simulink model "PIL_NO_RPI_new"  (R2021a)
settings: Solver=FixedStepAuto  StartTime=0.0  StopTime=60  FixedStep=0.001  RelTol=1e-3  EnableMultiTasking=on
values from neighbouring files (symbols this model uses):
  den_lpf_d = den_lpf20    [Mainframe_init.m]    (also in load_autopilot.m)
  Enable_Gyros = 0    [Mainframe_init.m]
  Enable_INS = 0    [Mainframe_init.m]
  num_lpf_d = num_lpf20    [Mainframe_init.m]    (also in load_autopilot.m)
undefined symbols (not defined in the file or in its folder): act_dmp, act_omega, Actuator, Aerodynamics, aMode, Autopilot, AUX, c_b_WGS, c_be, c_flat, c_grav, c_h_geop0, c_h_geope, c_pa0, c_pe, c_r0, c_rot, c_rsma, c_Tmp0, d_siB_0, d_siB_max, d_siB_min, dd_siB_max, dd_siB_min, dev, DiscIntNeverNeededParam, e_pa, e_Tmp, fin_maxrate, flag_I_act_switch, flag_I_aero_switch, flag_I_flat, flag_I_gravity_switch, flag_I_rot, h_bkpts_m, hcr, HIL_Data, JMMM_0, JMMM_e, JSPB_e, Ki_phi_vec, Kp_p_vec, Kp_phi_vec, lat_0, lon_0, Mass_Props, mB_0, mM_0, mM_e, National_Instruments, Newton, p, pBII_0, PCIe, phi, pMPB, pNPB, propellant_kg, prp_FBPB, prp_mdot ... (+40)
libraries: simulink x32, simulink_extras x23, aerolibcommonsys x4, pil_lib x2, custom_blocks x1, px4lib x1, sldrtlib x1, aerolibnav x1
(part 16 of 16)

== system PIL_NO_RPI_new/Non-linear Flight Dynamic Model1/Subsystem1/GRM_Airframe/motion_kinematics/calc_motion_kinematics/earth_rotation/quaternion_integration/Subsystem1/conjugate_quaternion1 ==
  note: Outputs [size]:
      |
      | q_conj [4]
  note: Inputs [size]:
      |
      | q [4]
  q : Inport
  Demux : Demux  Outputs=[3;1]
  Gain1 : Gain  Gain=-1
  Vector Concatenate : Concatenate
  q_conj : Outport  VectorParamsAs1DForOutWhenUnconnected=off
  wires:
  Demux/2 -> Vector Concatenate/2
  Gain1/1 -> Vector Concatenate/1
  Demux/1 -> Gain1/1
  Vector Concatenate/1 -> q_conj/1
  q/1 -> Demux/1

== system PIL_NO_RPI_new/Non-linear Flight Dynamic Model1/Subsystem1/GRM_Airframe/motion_kinematics/calc_motion_kinematics/earth_rotation/quaternion_integration/Subsystem1/conjugate_quaternion2 ==
  note: Outputs [size]:
      |
      | q_conj [4]
  note: Inputs [size]:
      |
      | q [4]
  q : Inport
  Demux : Demux  Outputs=[3;1]
  Gain1 : Gain  Gain=-1
  Vector Concatenate : Concatenate
  q_conj : Outport  VectorParamsAs1DForOutWhenUnconnected=off
  wires:
  Demux/2 -> Vector Concatenate/2
  Gain1/1 -> Vector Concatenate/1
  Demux/1 -> Gain1/1
  Vector Concatenate/1 -> q_conj/1
  q/1 -> Demux/1

== system PIL_NO_RPI_new/Non-linear Flight Dynamic Model1/Subsystem1/GRM_Airframe/motion_kinematics/calc_motion_kinematics/earth_rotation/quaternion_integration1/Subsystem1/conjugate_quaternion1 ==
  note: Outputs [size]:
      |
      | q_conj [4]
  note: Inputs [size]:
      |
      | q [4]
  q : Inport
  Demux : Demux  Outputs=[3;1]
  Gain1 : Gain  Gain=-1
  Vector Concatenate : Concatenate
  q_conj : Outport  VectorParamsAs1DForOutWhenUnconnected=off
  wires:
  Demux/2 -> Vector Concatenate/2
  Gain1/1 -> Vector Concatenate/1
  Demux/1 -> Gain1/1
  Vector Concatenate/1 -> q_conj/1
  q/1 -> Demux/1

== system PIL_NO_RPI_new/Non-linear Flight Dynamic Model1/Subsystem1/GRM_Airframe/motion_kinematics/calc_motion_kinematics/earth_rotation/quaternion_integration1/Subsystem1/conjugate_quaternion2 ==
  note: Outputs [size]:
      |
      | q_conj [4]
  note: Inputs [size]:
      |
      | q [4]
  q : Inport
  Demux : Demux  Outputs=[3;1]
  Gain1 : Gain  Gain=-1
  Vector Concatenate : Concatenate
  q_conj : Outport  VectorParamsAs1DForOutWhenUnconnected=off
  wires:
  Demux/2 -> Vector Concatenate/2
  Gain1/1 -> Vector Concatenate/1
  Demux/1 -> Gain1/1
  Vector Concatenate/1 -> q_conj/1
  q/1 -> Demux/1

== system PIL_NO_RPI_new/Non-linear Flight Dynamic Model1/Subsystem1/GRM_Airframe/rb_eom/eom_6dof/Rigid_Body_EOM_6_DOF/rb_eom_6dof/calc_d_qIB/conjugate_quaternion ==
  note: Outputs [size]:
      |
      | q_conj [4]
  note: Inputs [size]:
      |
      | q [4]
  q : Inport
  Demux : Demux  Outputs=[3;1]
  Gain1 : Gain  Gain=-1
  Vector Concatenate : Concatenate
  q_conj : Outport  VectorParamsAs1DForOutWhenUnconnected=off
  wires:
  Demux/2 -> Vector Concatenate/2
  Gain1/1 -> Vector Concatenate/1
  Demux/1 -> Gain1/1
  Vector Concatenate/1 -> q_conj/1
  q/1 -> Demux/1

== system PIL_NO_RPI_new/Non-linear Flight Dynamic Model1/Subsystem1/GRM_Airframe/rb_eom/eom_6dof/Rigid_Body_EOM_6_DOF/rb_eom_6dof/calc_d_qIB/conjugate_quaternion1 ==
  note: Outputs [size]:
      |
      | q_conj [4]
  note: Inputs [size]:
      |
      | q [4]
  q : Inport
  Demux : Demux  Outputs=[3;1]
  Gain1 : Gain  Gain=-1
  Vector Concatenate : Concatenate
  q_conj : Outport  VectorParamsAs1DForOutWhenUnconnected=off
  wires:
  Demux/2 -> Vector Concatenate/2
  Gain1/1 -> Vector Concatenate/1
  Demux/1 -> Gain1/1
  Vector Concatenate/1 -> q_conj/1
  q/1 -> Demux/1

== system PIL_NO_RPI_new/Non-linear Flight Dynamic Model1/Subsystem1/GRM_Airframe/aerodynamics/aerodynamic_via_lookup/calc_aero_for_mom/launch_rail/initial_altitude/trafo_E_to_geodetic/Geodetic_altitude ==
  pBEE : Inport
  c_rsma : Inport  Port=2
  c_flat : Inport  Port=3
  lat : Inport  Port=4
  Add : Sum
  Constant : Constant
  Gain : Gain  Gain=2
  Product : Product  Inputs=*/  InputSameDT=on  RndMeth=Zero  SaturateOnIntegerOverflow=on  OutDataTypeStr=Inherit: Same as first input
  Product1 : Product
  Product2 : Product
  Product3 : Product
  Product4 : Product  Inputs=*/  InputSameDT=on  RndMeth=Zero  SaturateOnIntegerOverflow=on  OutDataTypeStr=Inherit: Same as first input
  Product5 : Product  Inputs=3
  Selector : Selector  IndexMode=Zero-based  InputPortWidth=3  IndexOptions=Index vector (dialog)  Indices=0  OutputSizes=1
  Selector1 : Selector  IndexMode=Zero-based  InputPortWidth=3  IndexOptions=Index vector (dialog)  Indices=1  OutputSizes=1
  Sqrt : Sqrt  SaturateOnIntegerOverflow=on
  Sqrt1 : Sqrt  SaturateOnIntegerOverflow=on
  Subtract : Sum  Inputs=+-
  Subtract1 : Sum  Inputs=+-
  Sum : Sum  Inputs=+-  InputSameDT=on  SaturateOnIntegerOverflow=on  OutDataTypeStr=Inherit: Same as first input
  Trigonometric Function : Trigonometry
  cos(latGD) : Trigonometry  Operator=cos
  alt : Outport  VectorParamsAs1DForOutWhenUnconnected=off
  wires:
  Product4/1 -> Sum/2
  Trigonometric Function/1 -> Product5/1, Product5/2
  Product5/1 -> Subtract1/2
  Constant/1 -> Subtract1/1
  Subtract1/1 -> Sqrt1/1
  Sqrt1/1 -> Product4/2
  c_flat/1 -> Gain/1, Product3/2, Product3/1
  Gain/1 -> Subtract/1
  Product3/1 -> Subtract/2
  pBEE/1 -> Selector/1, Selector1/1
  Add/1 -> Sqrt/1
  Product2/1 -> Add/2
  Product1/1 -> Add/1
  Selector1/1 -> Product2/1, Product2/2
  Selector/1 -> Product1/1, Product1/2
  Sum/1 -> alt/1  "alt"
  Product/1 -> Sum/1
  Subtract/1 -> Product5/3
  c_rsma/1 -> Product4/1
  cos(latGD)/1 -> Product/2
  Sqrt/1 -> Product/1
  lat/1 -> cos(latGD)/1, Trigonometric Function/1

== system PIL_NO_RPI_new/Non-linear Flight Dynamic Model1/Subsystem1/GRM_Airframe/aerodynamics/aerodynamic_via_lookup/calc_aero_for_mom/launch_rail/initial_altitude/trafo_E_to_geodetic/Geodetic_latitude ==
  pBEE : Inport
  c_rsma : Inport  Port=2
  c_flat : Inport  Port=3
  Add : Sum
  Add1 : Sum
  Constant : Constant
  Demux1 : Demux  Outputs=[1;1;1]
      settings: DisplayOption=none
  Divide : Product  Inputs=*/
  Divide1 : Product  Inputs=*/
  Divide2 : Product  Inputs=*/
  Gain : Gain  Gain=2
  Product{,1..7} (8 alike) : Product
  Product{8..11} (4 alike) : Product  Inputs=3
  Sqrt : Sqrt  SaturateOnIntegerOverflow=on
  Subtract{,1..3} (4 alike) : Sum  Inputs=+-
  Trigonometric Function : Trigonometry  Operator=atan
  Trigonometric Function1 : Trigonometry  Operator=atan
  Trigonometric Function2 : Trigonometry
  Trigonometric Function3 : Trigonometry  Operator=cos
  lat : Outport  VectorParamsAs1DForOutWhenUnconnected=off
  wires:
  Divide/1 -> Product10/1
  Product9/1 -> Product11/3
  Product11/1 -> Subtract3/2
  Subtract3/1 -> Divide2/2
  Add1/1 -> Divide2/1
  Product10/1 -> Add1/2
  Product8/1 -> Product10/3
  Trigonometric Function3/1 -> Product9/1, Product9/3, Product9/2
  Trigonometric Function2/1 -> Product8/1, Product8/3, Product8/2
  Divide2/1 -> Trigonometric Function1/1
  Divide1/1 -> Trigonometric Function/1
  Product7/1 -> Divide1/2
  Product6/1 -> Divide1/1
  Subtract2/1 -> Divide/1
  Product5/1 -> Divide/2, Subtract2/2
  Product4/1 -> Subtract2/1
  Gain/1 -> Subtract1/1
  Product3/1 -> Subtract1/2
  Sqrt/1 -> [P]
  Add/1 -> Sqrt/1
  Product2/1 -> Add/2
  Product1/1 -> Add/1
  Product/1 -> [b]
  Subtract/1 -> Product/2
  Constant/1 -> Subtract/1
  Trigonometric Function1/1 -> lat/1  "lat"
  [a] -> Product11/2
  Subtract1/1 -> Product11/1
  [P] -> Subtract3/1
  [b] -> Product10/2
  [z] -> Add1/1
  [b] -> Product7/2
  [P] -> Product7/1
  Trigonometric Function/1 -> Trigonometric Function2/1, Trigonometric Function3/1
  [a] -> Product6/2
  [z] -> Product6/1
  [f] -> Gain/1, Product3/1, Product3/2
  [b] -> Product5/1, Product5/2
  [a] -> Product4/1, Product4/2
  Demux1/2 -> Product2/1, Product2/2
  Demux1/1 -> Product1/1, Product1/2
  [f] -> Subtract/2
  [a] -> Product/1
  Demux1/3 -> [z]
  pBEE/1 -> Demux1/1
  c_rsma/1 -> [a]
  c_flat/1 -> [f]

== system PIL_NO_RPI_new/Non-linear Flight Dynamic Model1/Subsystem1/GRM_Airframe/aerodynamics/aerodynamic_via_lookup/calc_aero_for_mom/launch_rail1/initial_altitude/trafo_E_to_geodetic/Geodetic_altitude ==
  pBEE : Inport
  c_rsma : Inport  Port=2
  c_flat : Inport  Port=3
  lat : Inport  Port=4
  Add : Sum
  Constant : Constant
  Gain : Gain  Gain=2
  Product : Product  Inputs=*/  InputSameDT=on  RndMeth=Zero  SaturateOnIntegerOverflow=on  OutDataTypeStr=Inherit: Same as first input
  Product1 : Product
  Product2 : Product
  Product3 : Product
  Product4 : Product  Inputs=*/  InputSameDT=on  RndMeth=Zero  SaturateOnIntegerOverflow=on  OutDataTypeStr=Inherit: Same as first input
  Product5 : Product  Inputs=3
  Selector : Selector  IndexMode=Zero-based  InputPortWidth=3  IndexOptions=Index vector (dialog)  Indices=0  OutputSizes=1
  Selector1 : Selector  IndexMode=Zero-based  InputPortWidth=3  IndexOptions=Index vector (dialog)  Indices=1  OutputSizes=1
  Sqrt : Sqrt  SaturateOnIntegerOverflow=on
  Sqrt1 : Sqrt  SaturateOnIntegerOverflow=on
  Subtract : Sum  Inputs=+-
  Subtract1 : Sum  Inputs=+-
  Sum : Sum  Inputs=+-  InputSameDT=on  SaturateOnIntegerOverflow=on  OutDataTypeStr=Inherit: Same as first input
  Trigonometric Function : Trigonometry
  cos(latGD) : Trigonometry  Operator=cos
  alt : Outport  VectorParamsAs1DForOutWhenUnconnected=off
  wires:
  Product4/1 -> Sum/2
  Trigonometric Function/1 -> Product5/1, Product5/2
  Product5/1 -> Subtract1/2
  Constant/1 -> Subtract1/1
  Subtract1/1 -> Sqrt1/1
  Sqrt1/1 -> Product4/2
  c_flat/1 -> Gain/1, Product3/2, Product3/1
  Gain/1 -> Subtract/1
  Product3/1 -> Subtract/2
  pBEE/1 -> Selector/1, Selector1/1
  Add/1 -> Sqrt/1
  Product2/1 -> Add/2
  Product1/1 -> Add/1
  Selector1/1 -> Product2/1, Product2/2
  Selector/1 -> Product1/1, Product1/2
  Sum/1 -> alt/1  "alt"
  Product/1 -> Sum/1
  Subtract/1 -> Product5/3
  c_rsma/1 -> Product4/1
  cos(latGD)/1 -> Product/2
  Sqrt/1 -> Product/1
  lat/1 -> cos(latGD)/1, Trigonometric Function/1

== system PIL_NO_RPI_new/Non-linear Flight Dynamic Model1/Subsystem1/GRM_Airframe/aerodynamics/aerodynamic_via_lookup/calc_aero_for_mom/launch_rail1/initial_altitude/trafo_E_to_geodetic/Geodetic_latitude ==
  pBEE : Inport
  c_rsma : Inport  Port=2
  c_flat : Inport  Port=3
  Add : Sum
  Add1 : Sum
  Constant : Constant
  Demux1 : Demux  Outputs=[1;1;1]
      settings: DisplayOption=none
  Divide : Product  Inputs=*/
  Divide1 : Product  Inputs=*/
  Divide2 : Product  Inputs=*/
  Gain : Gain  Gain=2
  Product{,1..7} (8 alike) : Product
  Product{8..11} (4 alike) : Product  Inputs=3
  Sqrt : Sqrt  SaturateOnIntegerOverflow=on
  Subtract{,1..3} (4 alike) : Sum  Inputs=+-
  Trigonometric Function : Trigonometry  Operator=atan
  Trigonometric Function1 : Trigonometry  Operator=atan
  Trigonometric Function2 : Trigonometry
  Trigonometric Function3 : Trigonometry  Operator=cos
  lat : Outport  VectorParamsAs1DForOutWhenUnconnected=off
  wires:
  Divide/1 -> Product10/1
  Product9/1 -> Product11/3
  Product11/1 -> Subtract3/2
  Subtract3/1 -> Divide2/2
  Add1/1 -> Divide2/1
  Product10/1 -> Add1/2
  Product8/1 -> Product10/3
  Trigonometric Function3/1 -> Product9/1, Product9/3, Product9/2
  Trigonometric Function2/1 -> Product8/1, Product8/3, Product8/2
  Divide2/1 -> Trigonometric Function1/1
  Divide1/1 -> Trigonometric Function/1
  Product7/1 -> Divide1/2
  Product6/1 -> Divide1/1
  Subtract2/1 -> Divide/1
  Product5/1 -> Divide/2, Subtract2/2
  Product4/1 -> Subtract2/1
  Gain/1 -> Subtract1/1
  Product3/1 -> Subtract1/2
  Sqrt/1 -> [P]
  Add/1 -> Sqrt/1
  Product2/1 -> Add/2
  Product1/1 -> Add/1
  Product/1 -> [b]
  Subtract/1 -> Product/2
  Constant/1 -> Subtract/1
  Trigonometric Function1/1 -> lat/1  "lat"
  [a] -> Product11/2
  Subtract1/1 -> Product11/1
  [P] -> Subtract3/1
  [b] -> Product10/2
  [z] -> Add1/1
  [b] -> Product7/2
  [P] -> Product7/1
  Trigonometric Function/1 -> Trigonometric Function2/1, Trigonometric Function3/1
  [a] -> Product6/2
  [z] -> Product6/1
  [f] -> Gain/1, Product3/1, Product3/2
  [b] -> Product5/1, Product5/2
  [a] -> Product4/1, Product4/2
  Demux1/2 -> Product2/1, Product2/2
  Demux1/1 -> Product1/1, Product1/2
  [f] -> Subtract/2
  [a] -> Product/1
  Demux1/3 -> [z]
  pBEE/1 -> Demux1/1
  c_rsma/1 -> [a]
  c_flat/1 -> [f]

== matlab function PIL_NO_RPI_new/Non-linear Flight Dynamic Model1/GRM_Airframe/fin_actuators/Rudder2/Limiting_Acceleration ==
  data: siB input; dd_siB_l output; d_siB input; dd_siB input; siB_min parameter; siB_max parameter; d_siB_min parameter; d_siB_max parameter; dd_siB_min parameter; dd_siB_max parameter
function dd_siB_l   = fcn(siB, d_siB, dd_siB, siB_min, siB_max, d_siB_min, d_siB_max, dd_siB_min, dd_siB_max)
%#codegen

%%   
dd_siB_l = dd_siB;

if dd_siB < dd_siB_min
    dd_siB_l = dd_siB_min;

elseif dd_siB_max < dd_siB
    dd_siB_l = dd_siB_max;
end;

if (siB <= siB_min && d_siB < 0) || (siB_max <= siB && 0 < d_siB)
    dd_siB_l = 0;
end;

if (d_siB <= d_siB_min && dd_siB < 0) || (d_siB_max <= d_siB && 0 < dd_siB)
    dd_siB_l = 0;
end

== matlab function PIL_NO_RPI_new/Non-linear Flight Dynamic Model1/GRM_Airframe/fin_actuators/Rudder2/Limiting_Rate ==
  data: siB input; d_siB_l output; d_siB input; siB_min parameter; siB_max parameter; d_siB_min parameter; d_siB_max parameter
function d_siB_l  = fcn(siB, d_siB, siB_min, siB_max, d_siB_min, d_siB_max)
%#codegen

%%  
d_siB_l = d_siB;

if d_siB < d_siB_min
    d_siB_l = d_siB_min;
    
elseif d_siB_max < d_siB
    d_siB_l = d_siB_max;
    
end

 if (siB <= siB_min && d_siB < 0) || (siB_max <= siB && 0 < d_siB)
    d_siB_l = 0;
 end

== matlab function PIL_NO_RPI_new/Non-linear Flight Dynamic Model1/GRM_Airframe/fin_actuators/Rudder3/Limiting_Acceleration ==
  data: siB input; dd_siB_l output; d_siB input; dd_siB input; siB_min parameter; siB_max parameter; d_siB_min parameter; d_siB_max parameter; dd_siB_min parameter; dd_siB_max parameter
function dd_siB_l   = fcn(siB, d_siB, dd_siB, siB_min, siB_max, d_siB_min, d_siB_max, dd_siB_min, dd_siB_max)
%#codegen

%%   
dd_siB_l = dd_siB;

if dd_siB < dd_siB_min
    dd_siB_l = dd_siB_min;

elseif dd_siB_max < dd_siB
    dd_siB_l = dd_siB_max;
end;

if (siB <= siB_min && d_siB < 0) || (siB_max <= siB && 0 < d_siB)
    dd_siB_l = 0;
end;

if (d_siB <= d_siB_min && dd_siB < 0) || (d_siB_max <= d_siB && 0 < dd_siB)
    dd_siB_l = 0;
end

== matlab function PIL_NO_RPI_new/Non-linear Flight Dynamic Model1/GRM_Airframe/fin_actuators/Rudder3/Limiting_Rate ==
  data: siB input; d_siB_l output; d_siB input; siB_min parameter; siB_max parameter; d_siB_min parameter; d_siB_max parameter
function d_siB_l  = fcn(siB, d_siB, siB_min, siB_max, d_siB_min, d_siB_max)
%#codegen

%%  
d_siB_l = d_siB;

if d_siB < d_siB_min
    d_siB_l = d_siB_min;
    
elseif d_siB_max < d_siB
    d_siB_l = d_siB_max;
    
end

 if (siB <= siB_min && d_siB < 0) || (siB_max <= siB && 0 < d_siB)
    d_siB_l = 0;
 end

== matlab function PIL_NO_RPI_new/Non-linear Flight Dynamic Model1/Subsystem1/Extract States/MATLAB Function1 ==
  data: q input; q_conj output
%% Computes the conjugate complex quaternion
%
% INPUTS:    
%   MANDATORY:
%    4x1    double   q           ....... quaternion
%    
% OUTPUTS:   
%    4x1    double   q_conj      ....... conjugated quaternion
%
% ABSTRACT: 
% This function computes teh conjugate complex quaternion
%
% DESCRIPTION: 
% This function computes teh conjugate complex quaternion
%
% PROJECT:
%        ***  ISim - Generic Interceptor Simulation ***
%
% CHANGE LOG
% Date          Name                Description         Version
% 2015/06/10    T. Z�belein         initial version     V 1.0 

%% 
function q_conj = conjq(q)
%#codegen

  q_conj    = -q;
  q_conj(4) =  q(4);

end

== matlab function PIL_NO_RPI_new/Non-linear Flight Dynamic Model1/Subsystem1/GRM_Airframe/aerodynamics/logic_base_drag/MATLAB Function ==
  data: u input; flag_base_drag output; t_prp2 input
function flag_base_drag = fcn(u, t_prp2)
%#codegen
if u >= 0 && u <= t_prp2 
    y = 0;
else
    y = 1;
    
end
flag_base_drag = y;

== matlab function PIL_NO_RPI_new/Non-linear Flight Dynamic Model1/Subsystem1/GRM_Airframe/environment/WGS84_Gravitation/WGS84_Gravity_Implementation ==
  data: pE input; lat_rad input; long_rad input; gamma_R output; c_rsma parameter; c_b_WGS parameter; c_grav parameter; c_rot parameter; flg_omega_enabled parameter
% Nach dem WGS84 Standard implementierte Gravitationsbeschleunigung 
%
% INPUTS:    
%   MANDATORY:
%       pE          ....... Positionsvektor im ECEF System
%       c_rsma      ....... Große Halbachse des WGS84 Ellipsoids
%       c_b_WGS     ....... Kleine Halbachse des WGS84 Ellipsoids
%       c_grav      ....... Gravitationskonstante der Erde nach WGS84
%       c_rot       ....... Rotationsgeschwindigkeit der Erde nach WGS84
%       flg_omega_enabled . Flag, die bestimmt ob die Rotation der Erde
%                           mitberechnet wird.
% 
% OUTPUTS:   
%       gamma_h     ....... Betrag des Gravitationsvektors
% 
% ABSTRACT: 
% Berechnet den absoluten Gravitationsbeschleunigungsbetrag nach Formel 4-4
% bis 4-13 des WGS84 Standards ( Technical Report
% "Department of Defense World Geodetic System 1984", NIMA TR8350.2,
% Third Edition, Amendment 1 vom 3 Januar 2000)
% 
%
% PROJECT:
%              *** GENERIC INTERCEPTOR SIMULATION ***
%
% REFERENCES:
% Technical Report
% "Department of Defense World Geodetic System 1984", NIMA TR8350.2,
% Third Edition, Amendment 1 vom 3 Januar 2000
%
% CHANGE LOG
% Date          Name                Description                     Version
% 2016.08.24    Philippe Petit      Inital Version                  V1.0
% 2016.11.16    Philippe Petit      Ausgabe der Gravitation als     V1.1
%                                   Vektor
% 2017.03.08    Christian Heise     Korrektur der Ausgabe, so dass  V1.2
%                                   wirklich ein Vektor im ECEF-
%                                   Frame zurückgegeben wird.

function gamma_R = wgs84_normalgravity(pE, lat_rad, long_rad, c_rsma, c_b_WGS, c_grav, c_rot, flg_omega_enabled)
%WGS84 Gravity Implementation
% a = 6378137.0;                  %[m], WGS84 Semi-major Axis 
% b = 6356752.3142;               %[m], WGS84 Semi-minor Axis
% omega = 7292115.8553e-11;       %[rad/s], WGS84 Angular Velocity of the Earth
% GM = 3986004.418e8;             %[m^3/s^2], Earths, Gravitational Constant
a       = c_rsma;
b       = c_b_WGS;
omega   = c_rot;
GM      = c_grav;
phi     = lat_rad;
lambda  = long_rad;

if norm(pE) < b
    error('Radius kleiner als die kleine halbachse...')
end

%Parse den Positionsvektor
x = pE(1);
y = pE(2);
z = pE(3);

%Formel 4-7 bis 4-13
E       = sqrt(a^2 - b^2);
u       = sqrt(1/2*(x^2+y^2+z^2-E^2)*(1+sqrt( 1 + (4*E^2*z^2)/(x^2+y^2+z^2-E^2)^2) ) );
beta    = atan2( z*sqrt(u^2+E^2) , u*sqrt(x^2+y^2) );
w       = sqrt((u^2 + E^2*sin(beta)^2)/(u^2 + E^2));
q       = 1/2*((1+3*u^2/E^2)*atan2(E,u)-3*u/E);
q_0     = 1/2*((1+3*b^2/E^2)*atan2(E,b)-3*b/E);
q_dash  = 3*(1+u^2/E^2)*(1-u/E*atan2(E,u))-1;

%Formel 4-5 und 4-6
gamma_u     = -1/w*( GM/(u^2+E^2) + omega^2*a^2*E/(u^2 + E^2)*q_dash/q_0*(1/2*sin(beta)^2 - 1/6) ) + flg_omega_enabled*1/w*omega^2*u*cos(beta)^2;
gamma_beta  = 1/w*omega^2*a^2/(u^2 + E^2)*q/q_0*sin(beta)*cos(beta) - flg_omega_enabled*1/w*omega^2*sqrt(u^2 + E^2) *sin(beta)*cos(beta);
gamma_lambda = 0;

%Formel 4-18 & 4-19
R1  = [u/(w*sqrt(u^2 + E^2))*cos(beta)*cos(lambda), -1/w*sin(beta)*cos(lambda), -sin(lambda);...                                      %Element(1,3)
       u/(w*sqrt(u^2 + E^2))*cos(beta)*sin(lambda), -1/w*sin(beta)*sin(lambda),  cos(lambda);...
       1/w*sin(beta)                              , u/(w*sqrt(u^2 + E^2))*cos(beta), 0];
% R2  = [cos(phi)*cos(lambda), cos(phi)*sin(lambda), sin(phi);...
%       -sin(phi)*cos(lambda), -sin(phi)*sin(lambda), cos(phi);...
%       -sin(lambda), cos(lambda), 0];
  
%Formel 4-16
gamma_E = [gamma_u; gamma_beta; gamma_lambda];
gamma_R = R1*gamma_E;

== matlab function PIL_NO_RPI_new/Non-linear Flight Dynamic Model1/Subsystem1/GRM_Airframe/fin_actuators/Rudder/Limiting_Acceleration ==
  data: siB input; dd_siB_l output; d_siB input; dd_siB input; siB_min parameter; siB_max parameter; d_siB_min parameter; d_siB_max parameter; dd_siB_min parameter; dd_siB_max parameter
function dd_siB_l   = fcn(siB, d_siB, dd_siB, siB_min, siB_max, d_siB_min, d_siB_max, dd_siB_min, dd_siB_max)
%#codegen

%%   
dd_siB_l = dd_siB;

if dd_siB < dd_siB_min
    dd_siB_l = dd_siB_min;

elseif dd_siB_max < dd_siB
    dd_siB_l = dd_siB_max;
end;

if (siB <= siB_min && d_siB < 0) || (siB_max <= siB && 0 < d_siB)
    dd_siB_l = 0;
end;

if (d_siB <= d_siB_min && dd_siB < 0) || (d_siB_max <= d_siB && 0 < dd_siB)
    dd_siB_l = 0;
end

== matlab function PIL_NO_RPI_new/Non-linear Flight Dynamic Model1/Subsystem1/GRM_Airframe/fin_actuators/Rudder/Limiting_Rate ==
  data: siB input; d_siB_l output; d_siB input; siB_min parameter; siB_max parameter; d_siB_min parameter; d_siB_max parameter
function d_siB_l  = fcn(siB, d_siB, siB_min, siB_max, d_siB_min, d_siB_max)
%#codegen

%%  
d_siB_l = d_siB;

if d_siB < d_siB_min
    d_siB_l = d_siB_min;
    
elseif d_siB_max < d_siB
    d_siB_l = d_siB_max;
    
end

 if (siB <= siB_min && d_siB < 0) || (siB_max <= siB && 0 < d_siB)
    d_siB_l = 0;
 end

== matlab function PIL_NO_RPI_new/Non-linear Flight Dynamic Model1/Subsystem1/GRM_Airframe/fin_actuators/Rudder1/Limiting_Acceleration ==
  data: siB input; dd_siB_l output; d_siB input; dd_siB input; siB_min parameter; siB_max parameter; d_siB_min parameter; d_siB_max parameter; dd_siB_min parameter; dd_siB_max parameter
function dd_siB_l   = fcn(siB, d_siB, dd_siB, siB_min, siB_max, d_siB_min, d_siB_max, dd_siB_min, dd_siB_max)
%#codegen

%%   
dd_siB_l = dd_siB;

if dd_siB < dd_siB_min
    dd_siB_l = dd_siB_min;

elseif dd_siB_max < dd_siB
    dd_siB_l = dd_siB_max;
end;

if (siB <= siB_min && d_siB < 0) || (siB_max <= siB && 0 < d_siB)
    dd_siB_l = 0;
end;

if (d_siB <= d_siB_min && dd_siB < 0) || (d_siB_max <= d_siB && 0 < dd_siB)
    dd_siB_l = 0;
end

== matlab function PIL_NO_RPI_new/Non-linear Flight Dynamic Model1/Extract States/MATLAB Function1 ==
  data: q input; q_conj output
%% Computes the conjugate complex quaternion
%
% INPUTS:    
%   MANDATORY:
%    4x1    double   q           ....... quaternion
%    
% OUTPUTS:   
%    4x1    double   q_conj      ....... conjugated quaternion
%
% ABSTRACT: 
% This function computes teh conjugate complex quaternion
%
% DESCRIPTION: 
% This function computes teh conjugate complex quaternion
%
% PROJECT:
%        ***  ISim - Generic Interceptor Simulation ***
%
% CHANGE LOG
% Date          Name                Description         Version
% 2015/06/10    T. Z�belein         initial version     V 1.0 

%% 
function q_conj = conjq(q)
%#codegen

  q_conj    = -q;
  q_conj(4) =  q(4);

end

== matlab function PIL_NO_RPI_new/Non-linear Flight Dynamic Model1/Subsystem1/GRM_Airframe/fin_actuators/Rudder1/Limiting_Rate ==
  data: siB input; d_siB_l output; d_siB input; siB_min parameter; siB_max parameter; d_siB_min parameter; d_siB_max parameter
function d_siB_l  = fcn(siB, d_siB, siB_min, siB_max, d_siB_min, d_siB_max)
%#codegen

%%  
d_siB_l = d_siB;

if d_siB < d_siB_min
    d_siB_l = d_siB_min;
    
elseif d_siB_max < d_siB
    d_siB_l = d_siB_max;
    
end

 if (siB <= siB_min && d_siB < 0) || (siB_max <= siB && 0 < d_siB)
    d_siB_l = 0;
 end

== matlab function PIL_NO_RPI_new/Non-linear Flight Dynamic Model1/Subsystem1/GRM_Airframe/fin_actuators/Rudder2/Limiting_Acceleration ==
  data: siB input; dd_siB_l output; d_siB input; dd_siB input; siB_min parameter; siB_max parameter; d_siB_min parameter; d_siB_max parameter; dd_siB_min parameter; dd_siB_max parameter
function dd_siB_l   = fcn(siB, d_siB, dd_siB, siB_min, siB_max, d_siB_min, d_siB_max, dd_siB_min, dd_siB_max)
%#codegen

%%   
dd_siB_l = dd_siB;

if dd_siB < dd_siB_min
    dd_siB_l = dd_siB_min;

elseif dd_siB_max < dd_siB
    dd_siB_l = dd_siB_max;
end;

if (siB <= siB_min && d_siB < 0) || (siB_max <= siB && 0 < d_siB)
    dd_siB_l = 0;
end;

if (d_siB <= d_siB_min && dd_siB < 0) || (d_siB_max <= d_siB && 0 < dd_siB)
    dd_siB_l = 0;
end

== matlab function PIL_NO_RPI_new/Non-linear Flight Dynamic Model1/Subsystem1/GRM_Airframe/fin_actuators/Rudder2/Limiting_Rate ==
  data: siB input; d_siB_l output; d_siB input; siB_min parameter; siB_max parameter; d_siB_min parameter; d_siB_max parameter
function d_siB_l  = fcn(siB, d_siB, siB_min, siB_max, d_siB_min, d_siB_max)
%#codegen

%%  
d_siB_l = d_siB;

if d_siB < d_siB_min
    d_siB_l = d_siB_min;
    
elseif d_siB_max < d_siB
    d_siB_l = d_siB_max;
    
end

 if (siB <= siB_min && d_siB < 0) || (siB_max <= siB && 0 < d_siB)
    d_siB_l = 0;
 end

== matlab function PIL_NO_RPI_new/Non-linear Flight Dynamic Model1/Subsystem1/GRM_Airframe/fin_actuators/Rudder3/Limiting_Acceleration ==
  data: siB input; dd_siB_l output; d_siB input; dd_siB input; siB_min parameter; siB_max parameter; d_siB_min parameter; d_siB_max parameter; dd_siB_min parameter; dd_siB_max parameter
function dd_siB_l   = fcn(siB, d_siB, dd_siB, siB_min, siB_max, d_siB_min, d_siB_max, dd_siB_min, dd_siB_max)
%#codegen

%%   
dd_siB_l = dd_siB;

if dd_siB < dd_siB_min
    dd_siB_l = dd_siB_min;

elseif dd_siB_max < dd_siB
    dd_siB_l = dd_siB_max;
end;

if (siB <= siB_min && d_siB < 0) || (siB_max <= siB && 0 < d_siB)
    dd_siB_l = 0;
end;

if (d_siB <= d_siB_min && dd_siB < 0) || (d_siB_max <= d_siB && 0 < dd_siB)
    dd_siB_l = 0;
end

== matlab function PIL_NO_RPI_new/Non-linear Flight Dynamic Model1/Subsystem1/GRM_Airframe/fin_actuators/Rudder3/Limiting_Rate ==
  data: siB input; d_siB_l output; d_siB input; siB_min parameter; siB_max parameter; d_siB_min parameter; d_siB_max parameter
function d_siB_l  = fcn(siB, d_siB, siB_min, siB_max, d_siB_min, d_siB_max)
%#codegen

%%  
d_siB_l = d_siB;

if d_siB < d_siB_min
    d_siB_l = d_siB_min;
    
elseif d_siB_max < d_siB
    d_siB_l = d_siB_max;
    
end

 if (siB <= siB_min && d_siB < 0) || (siB_max <= siB && 0 < d_siB)
    d_siB_l = 0;
 end

== matlab function PIL_NO_RPI_new/Non-linear Flight Dynamic Model1/GRM_Airframe/aerodynamics/logic_base_drag/MATLAB Function ==
  data: u input; flag_base_drag output; t_prp2 input
function flag_base_drag = fcn(u, t_prp2)
%#codegen
if u >= 0 && u <= t_prp2 
    y = 0;
else
    y = 1;
    
end
flag_base_drag = y;

== matlab function PIL_NO_RPI_new/Non-linear Flight Dynamic Model1/GRM_Airframe/environment/WGS84_Gravitation/WGS84_Gravity_Implementation ==
  data: pE input; lat_rad input; long_rad input; gamma_R output; c_rsma parameter; c_b_WGS parameter; c_grav parameter; c_rot parameter; flg_omega_enabled parameter
% Nach dem WGS84 Standard implementierte Gravitationsbeschleunigung 
%
% INPUTS:    
%   MANDATORY:
%       pE          ....... Positionsvektor im ECEF System
%       c_rsma      ....... Große Halbachse des WGS84 Ellipsoids
%       c_b_WGS     ....... Kleine Halbachse des WGS84 Ellipsoids
%       c_grav      ....... Gravitationskonstante der Erde nach WGS84
%       c_rot       ....... Rotationsgeschwindigkeit der Erde nach WGS84
%       flg_omega_enabled . Flag, die bestimmt ob die Rotation der Erde
%                           mitberechnet wird.
% 
% OUTPUTS:   
%       gamma_h     ....... Betrag des Gravitationsvektors
% 
% ABSTRACT: 
% Berechnet den absoluten Gravitationsbeschleunigungsbetrag nach Formel 4-4
% bis 4-13 des WGS84 Standards ( Technical Report
% "Department of Defense World Geodetic System 1984", NIMA TR8350.2,
% Third Edition, Amendment 1 vom 3 Januar 2000)
% 
%
% PROJECT:
%              *** GENERIC INTERCEPTOR SIMULATION ***
%
% REFERENCES:
% Technical Report
% "Department of Defense World Geodetic System 1984", NIMA TR8350.2,
% Third Edition, Amendment 1 vom 3 Januar 2000
%
% CHANGE LOG
% Date          Name                Description                     Version
% 2016.08.24    Philippe Petit      Inital Version                  V1.0
% 2016.11.16    Philippe Petit      Ausgabe der Gravitation als     V1.1
%                                   Vektor
% 2017.03.08    Christian Heise     Korrektur der Ausgabe, so dass  V1.2
%                                   wirklich ein Vektor im ECEF-
%                                   Frame zurückgegeben wird.

function gamma_R = wgs84_normalgravity(pE, lat_rad, long_rad, c_rsma, c_b_WGS, c_grav, c_rot, flg_omega_enabled)
%WGS84 Gravity Implementation
% a = 6378137.0;                  %[m], WGS84 Semi-major Axis 
% b = 6356752.3142;               %[m], WGS84 Semi-minor Axis
% omega = 7292115.8553e-11;       %[rad/s], WGS84 Angular Velocity of the Earth
% GM = 3986004.418e8;             %[m^3/s^2], Earths, Gravitational Constant
a       = c_rsma;
b       = c_b_WGS;
omega   = c_rot;
GM      = c_grav;
phi     = lat_rad;
lambda  = long_rad;

if norm(pE) < b
    error('Radius kleiner als die kleine halbachse...')
end

%Parse den Positionsvektor
x = pE(1);
y = pE(2);
z = pE(3);

%Formel 4-7 bis 4-13
E       = sqrt(a^2 - b^2);
u       = sqrt(1/2*(x^2+y^2+z^2-E^2)*(1+sqrt( 1 + (4*E^2*z^2)/(x^2+y^2+z^2-E^2)^2) ) );
beta    = atan2( z*sqrt(u^2+E^2) , u*sqrt(x^2+y^2) );
w       = sqrt((u^2 + E^2*sin(beta)^2)/(u^2 + E^2));
q       = 1/2*((1+3*u^2/E^2)*atan2(E,u)-3*u/E);
q_0     = 1/2*((1+3*b^2/E^2)*atan2(E,b)-3*b/E);
q_dash  = 3*(1+u^2/E^2)*(1-u/E*atan2(E,u))-1;

%Formel 4-5 und 4-6
gamma_u     = -1/w*( GM/(u^2+E^2) + omega^2*a^2*E/(u^2 + E^2)*q_dash/q_0*(1/2*sin(beta)^2 - 1/6) ) + flg_omega_enabled*1/w*omega^2*u*cos(beta)^2;
gamma_beta  = 1/w*omega^2*a^2/(u^2 + E^2)*q/q_0*sin(beta)*cos(beta) - flg_omega_enabled*1/w*omega^2*sqrt(u^2 + E^2) *sin(beta)*cos(beta);
gamma_lambda = 0;

%Formel 4-18 & 4-19
R1  = [u/(w*sqrt(u^2 + E^2))*cos(beta)*cos(lambda), -1/w*sin(beta)*cos(lambda), -sin(lambda);...                                      %Element(1,3)
       u/(w*sqrt(u^2 + E^2))*cos(beta)*sin(lambda), -1/w*sin(beta)*sin(lambda),  cos(lambda);...
       1/w*sin(beta)                              , u/(w*sqrt(u^2 + E^2))*cos(beta), 0];
% R2  = [cos(phi)*cos(lambda), cos(phi)*sin(lambda), sin(phi);...
%       -sin(phi)*cos(lambda), -sin(phi)*sin(lambda), cos(phi);...
%       -sin(lambda), cos(lambda), 0];
  
%Formel 4-16
gamma_E = [gamma_u; gamma_beta; gamma_lambda];
gamma_R = R1*gamma_E;

== matlab function PIL_NO_RPI_new/Non-linear Flight Dynamic Model1/GRM_Airframe/fin_actuators/Rudder/Limiting_Acceleration ==
  data: siB input; dd_siB_l output; d_siB input; dd_siB input; siB_min parameter; siB_max parameter; d_siB_min parameter; d_siB_max parameter; dd_siB_min parameter; dd_siB_max parameter
function dd_siB_l   = fcn(siB, d_siB, dd_siB, siB_min, siB_max, d_siB_min, d_siB_max, dd_siB_min, dd_siB_max)
%#codegen

%%   
dd_siB_l = dd_siB;

if dd_siB < dd_siB_min
    dd_siB_l = dd_siB_min;

elseif dd_siB_max < dd_siB
    dd_siB_l = dd_siB_max;
end;

if (siB <= siB_min && d_siB < 0) || (siB_max <= siB && 0 < d_siB)
    dd_siB_l = 0;
end;

if (d_siB <= d_siB_min && dd_siB < 0) || (d_siB_max <= d_siB && 0 < dd_siB)
    dd_siB_l = 0;
end

== matlab function PIL_NO_RPI_new/Non-linear Flight Dynamic Model1/GRM_Airframe/fin_actuators/Rudder/Limiting_Rate ==
  data: siB input; d_siB_l output; d_siB input; siB_min parameter; siB_max parameter; d_siB_min parameter; d_siB_max parameter
function d_siB_l  = fcn(siB, d_siB, siB_min, siB_max, d_siB_min, d_siB_max)
%#codegen

%%  
d_siB_l = d_siB;

if d_siB < d_siB_min
    d_siB_l = d_siB_min;
    
elseif d_siB_max < d_siB
    d_siB_l = d_siB_max;
    
end

 if (siB <= siB_min && d_siB < 0) || (siB_max <= siB && 0 < d_siB)
    d_siB_l = 0;
 end

== matlab function PIL_NO_RPI_new/Non-linear Flight Dynamic Model1/GRM_Airframe/fin_actuators/Rudder1/Limiting_Acceleration ==
  data: siB input; dd_siB_l output; d_siB input; dd_siB input; siB_min parameter; siB_max parameter; d_siB_min parameter; d_siB_max parameter; dd_siB_min parameter; dd_siB_max parameter
function dd_siB_l   = fcn(siB, d_siB, dd_siB, siB_min, siB_max, d_siB_min, d_siB_max, dd_siB_min, dd_siB_max)
%#codegen

%%   
dd_siB_l = dd_siB;

if dd_siB < dd_siB_min
    dd_siB_l = dd_siB_min;

elseif dd_siB_max < dd_siB
    dd_siB_l = dd_siB_max;
end;

if (siB <= siB_min && d_siB < 0) || (siB_max <= siB && 0 < d_siB)
    dd_siB_l = 0;
end;

if (d_siB <= d_siB_min && dd_siB < 0) || (d_siB_max <= d_siB && 0 < dd_siB)
    dd_siB_l = 0;
end

== matlab function PIL_NO_RPI_new/Non-linear Flight Dynamic Model1/GRM_Airframe/fin_actuators/Rudder1/Limiting_Rate ==
  data: siB input; d_siB_l output; d_siB input; siB_min parameter; siB_max parameter; d_siB_min parameter; d_siB_max parameter
function d_siB_l  = fcn(siB, d_siB, siB_min, siB_max, d_siB_min, d_siB_max)
%#codegen

%%  
d_siB_l = d_siB;

if d_siB < d_siB_min
    d_siB_l = d_siB_min;
    
elseif d_siB_max < d_siB
    d_siB_l = d_siB_max;
    
end

 if (siB <= siB_min && d_siB < 0) || (siB_max <= siB && 0 < d_siB)
    d_siB_l = 0;
 end
